simulink model "FCHEV_mpc"  (R2023a)
settings: Solver=ode23tb  StartTime=0.0  StopTime=20e3  MaxStep=1e-1  RelTol=1e-6
values from neighbouring files (symbols this model uses):
  ds = 10    [init_mpc.m]
  P = 20    [init_mpc.m]
  Ts = 1    [init_mpc.m]
libraries: component_lib x15, mpclib x1
settings Model: Creator=maxjo65  LastModifiedBy=maxjo65
settings OptimizationCC: ReuseModelBlockBuffer=off
settings DebuggingCC: UnconnectedInputMsg=warning  UnconnectedOutputMsg=warning  UnconnectedLineMsg=warning
settings ModelReferenceCC: EnableRefExpFcnMdlSchedulingChecks=on
settings RTWCC: DLArmComputeVersion=19.05

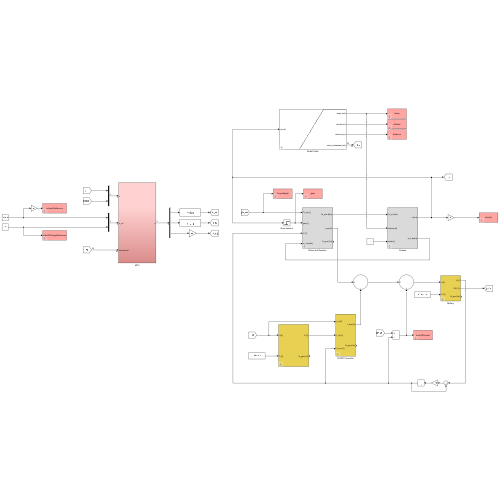
[thumbnail: Simulink's stored preview of the top-level diagram]
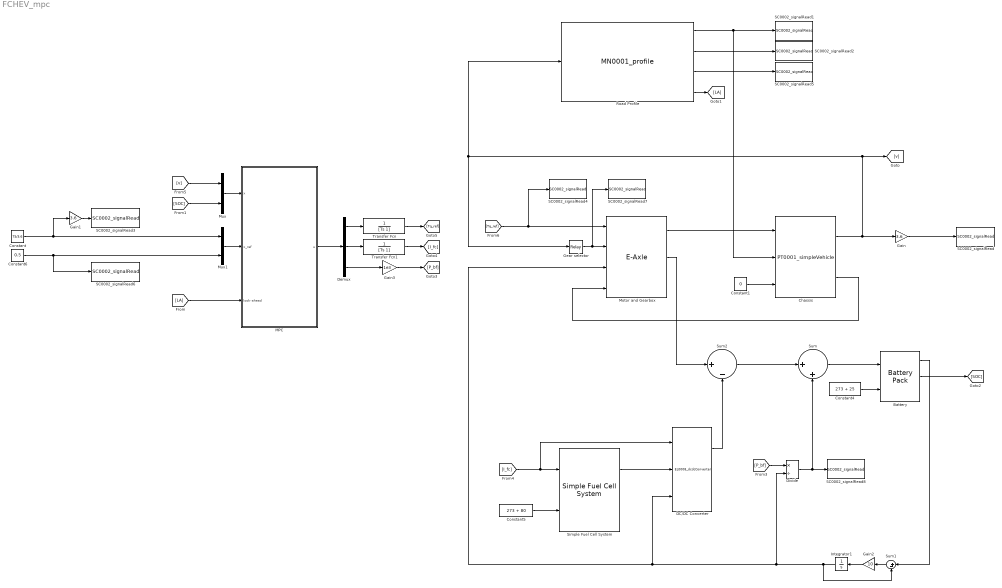
== system FCHEV_mpc ==
  Battery : component_lib/Battery Pack  SOC_0=0.5  Nx=60  Ny=180
  Chassis : component_lib/Powertrain/PT0001_simpleVehicle  m=40e3  r_w=0.5  A_f=10  C_d=0.5  rho_air=1.225  c_r0=0.0060  c_r1=2.3e-7  gain=600  v0=75/3.6  x0=0
  Constant : Constant  Value=75/3.6
  Constant1 : Constant  Value=0
  Constant4 : Constant  Value=273 + 25
  Constant5 : Constant  Value=273 + 80
  Constant6 : Constant  Value=0.5
  DC/DC Converter : component_lib/Electrochemistry/EL0008_dcdcConverter  eta_up=0.99  eta_down=0.99
  Demux : Demux  Outputs=3
  Divide : Product  Inputs=*/
  Gain : Gain  Gain=3.6
  Gain1 : Gain  Gain=3.6
  Gain2 : Gain  Gain=10
  Gain3 : Gain  Gain=1e3
  Gear selector : Relay  OnSwitchValue=30  OffSwitchValue=10  OnOutputValue=4  OffOutputValue=3
  Integrator1 : Integrator  InitialCondition=700
  MPC : Subsystem
  Motor and Gearbox : component_lib/E-Axle  n=3  V_nom=700
  Mux : Mux  Inputs=2
  Mux1 : Mux  Inputs=2
  Road Profile : component_lib/Mission/MN0001_profile  profile=incline.mat  x0=0  N_lookahead=P
  SC0002_signalRead : component_lib/Data & Control/SC0002_signalRead  SigName=velocity
  SC0002_signalRead1 : component_lib/Data & Control/SC0002_signalRead  SigName=slope
  SC0002_signalRead2 : component_lib/Data & Control/SC0002_signalRead  SigName=altitude
  SC0002_signalRead3 : component_lib/Data & Control/SC0002_signalRead  SigName=velocityReference
  SC0002_signalRead4 : component_lib/Data & Control/SC0002_signalRead  SigName=torqueSignal
  SC0002_signalRead5 : component_lib/Data & Control/SC0002_signalRead  SigName=distance
  SC0002_signalRead6 : component_lib/Data & Control/SC0002_signalRead  SigName=stateOfChargeReference
  SC0002_signalRead7 : component_lib/Data & Control/SC0002_signalRead  SigName=gear
  SC0002_signalRead8 : component_lib/Data & Control/SC0002_signalRead  SigName=burnOffCurrent
  Simple Fuel Cell System : component_lib/Simple Fuel Cell System  n_st=2  n=375
  Sum : Sum  Inputs=|++
  Sum1 : Sum  Inputs=|+-
  Sum2 : Sum  Inputs=|+-
  Transfer Fcn : TransferFcn  Denominator=[Ts 1]
  Transfer Fcn1 : TransferFcn  Denominator=[Ts 1]
  wires:
  Road Profile/1 -> SC0002_signalRead1/1, Chassis/2
  Gain/1 -> SC0002_signalRead/1
  Road Profile/2 -> SC0002_signalRead2/1
  Gain1/1 -> SC0002_signalRead3/1
  Constant1/1 -> Chassis/3
  Road Profile/4 -> [LA]
  Constant/1 -> Gain1/1, Mux1/1
  Motor and Gearbox/1 -> Chassis/1
  Chassis/2 -> Motor and Gearbox/4
  Chassis/1 -> Gear selector/1, Road Profile/1, [v], Gain/1
  Gear selector/1 -> SC0002_signalRead7/1, Motor and Gearbox/2
  Road Profile/3 -> SC0002_signalRead5/1
  Battery/1 -> Sum1/1
  Constant4/1 -> Battery/2
  Sum1/1 -> Gain2/1
  Gain2/1 -> Integrator1/1
  DC/DC Converter/1 -> Sum2/2
  Motor and Gearbox/2 -> Sum2/1
  Simple Fuel Cell System/1 -> DC/DC Converter/2
  Constant5/1 -> Simple Fuel Cell System/2
  Integrator1/1 -> Motor and Gearbox/3, DC/DC Converter/3, Divide/2, Sum1/2
  Battery/2 -> [SOC]
  Constant6/1 -> Mux1/2, SC0002_signalRead6/1
  Sum2/1 -> Sum/1
  Sum/1 -> Battery/1
  Divide/1 -> Sum/2, SC0002_signalRead8/1
  [P_bf] -> Divide/1
  [SOC] -> Mux/2
  MPC/1(u) -> Demux/1
  Demux/3 -> Gain3/1
  Gain3/1 -> [P_bf]
  Mux/1 -> MPC/1(x)
  Mux1/1 -> MPC/2(x_ref)
  [LA] -> MPC/3(look-ahead)
  [I_fc] -> DC/DC Converter/1, Simple Fuel Cell System/1
  [Tq_ref] -> SC0002_signalRead4/1, Motor and Gearbox/1
  [v] -> Mux/1
  Demux/2 -> Transfer Fcn1/1
  Demux/1 -> Transfer Fcn/1
  Transfer Fcn/1 -> [Tq_ref]
  Transfer Fcn1/1 -> [I_fc]

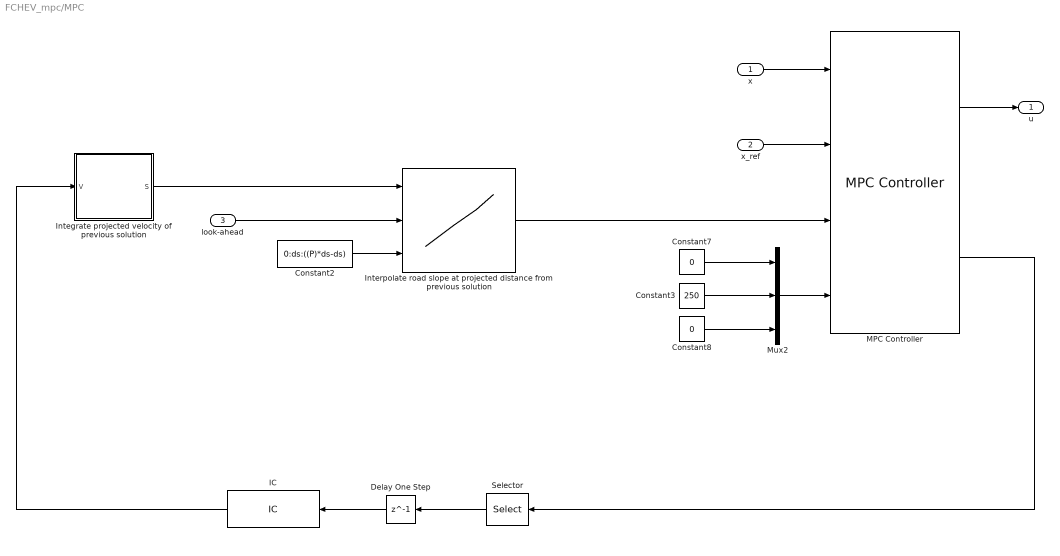
== system FCHEV_mpc/MPC ==
  x : Inport
  x_ref : Inport  Port=2
  look-ahead : Inport  Port=3
  Constant2 : Constant  Value=0:ds:((P)*ds-ds)
  Constant3 : Constant  Value=250
  Constant7 : Constant  Value=0
  Constant8 : Constant  Value=0
  Delay One Step : Delay  DelayLength=1
  IC : InitialCondition  Value=ones(P,1) * 75/3.6
  Integrate projected velocity of previous solution : MATLAB Function  TreatAsAtomicUnit=on
  Interpolate road slope at projected distance from previous solution : Lookup_n-D  NumberOfTableDimensions=1  BreakpointsForDimension1Source=Input port  BreakpointsForDimension1=[-5:5]  TableSource=Input port  Table=tanh([-5:5])  InternalRulePriority=Speed  RndMeth=Simplest
      settings: InputPortMap=u0,p221,p5
  MPC Controller : mpclib/MPC Controller  SCDEnableBlockLinearizationSpecification=on  mpcobj=mpcobj  is_multiple=0  enable_value=0  return_u0=off  updateMPCinCallerWorkspace=on  md_inport=on  mv_inport=off  uref_inport=on  return_cost=off  return_mvseq=off  return_qpstatus=off  return_xseq=on  return_state=off  return_ovseq=off  state_inport=off  umin_inport=off  umax_inport=off  ymin_inport=off  ymax_inport=off  cc_inport=off  ywt_inport=off  uwt_inport=off  duwt_inport=off  rhoeps_inport=off  pm_inport=off  MaximumP=10  HorizonChoice=FixedHorizon  n_ts=1  n_p=20  n_mv=3  n_md=1  n_ud=0  n_mo=2  n_uo=0  BlockDataType=double  SampleTimeInherited=off  switch_inport=off
  Mux2 : Mux  Inputs=3
  Selector : Selector  NumberOfDimensions=2  InputPortWidth=3  IndexOptions=Index vector (dialog),Index vector (dialog)  Indices=2:(P+1),1  OutputSizes=1,1
  u : Outport
  wires:
  Interpolate road slope at projected distance from previous solution/1 -> MPC Controller/3
  Mux2/1 -> MPC Controller/4
  x_ref/1 -> MPC Controller/2
  x/1 -> MPC Controller/1
  Integrate projected velocity of previous solution/1(S) -> Interpolate road slope at projected distance from previous solution/1
  MPC Controller/2 -> Selector/1
  Constant2/1 -> Interpolate road slope at projected distance from previous solution/3
  Constant7/1 -> Mux2/1
  Delay One Step/1 -> IC/1
  Selector/1 -> Delay One Step/1
  IC/1 -> Integrate projected velocity of previous solution/1(V)
  MPC Controller/1 -> u/1
  Constant3/1 -> Mux2/2
  Constant8/1 -> Mux2/3
  look-ahead/1 -> Interpolate road slope at projected distance from previous solution/2

== matlab function FCHEV_mpc/MPC/Integrate projected velocity of previous solution ==
  data: V input; S output; P parameter; Ts parameter
function S = fcn(V, P, Ts)

S = cumtrapz( (0:(P-1)) .* Ts, V);
